simulink model "Advance_Battery_Cooling"  (R2021a)
settings: Solver=FixedStepAuto  StartTime=0.0  StopTime=1400  FixedStep=1  RelTol=1e-3
values from neighbouring files (symbols this model uses):
  Bc = 810.5328    [Battery_Cooling.m]
  c = 1350    [Battery_Cooling.m]
  Cell_length = 0.227    [Battery_Cooling.m]
  cell_volatge = Cell(:,2:3)    [Battery_Cooling.m]
  Cell_Width = 0.226    [Battery_Cooling.m]
  Cr = [0.0117,0.0085,0.0090 ... (first row only)    [Battery_Cooling.m]
  h_conv = 5    [Battery_Cooling.m]
  m_flow_air = BCP/(1350*(20.15-BPT_max))    [Battery_Cooling.m]
  Mb = 150.2    [Battery_Cooling.m]
  Np = 2    [Battery_Cooling.m]
  Ns = 96    [Battery_Cooling.m]
  Ri = 0.0023    [Battery_Cooling.m]
  SOC = [0;0.1;0.25;0.5;0.75;0.9;1]    [Battery_Cooling.m]
  T = [278.15;293.15;313.15]    [Battery_Cooling.m]
  Tamb = 293.15    [Battery_Cooling.m]
settings Model: Creator=LENOVO  LastModifiedBy=LENOVO

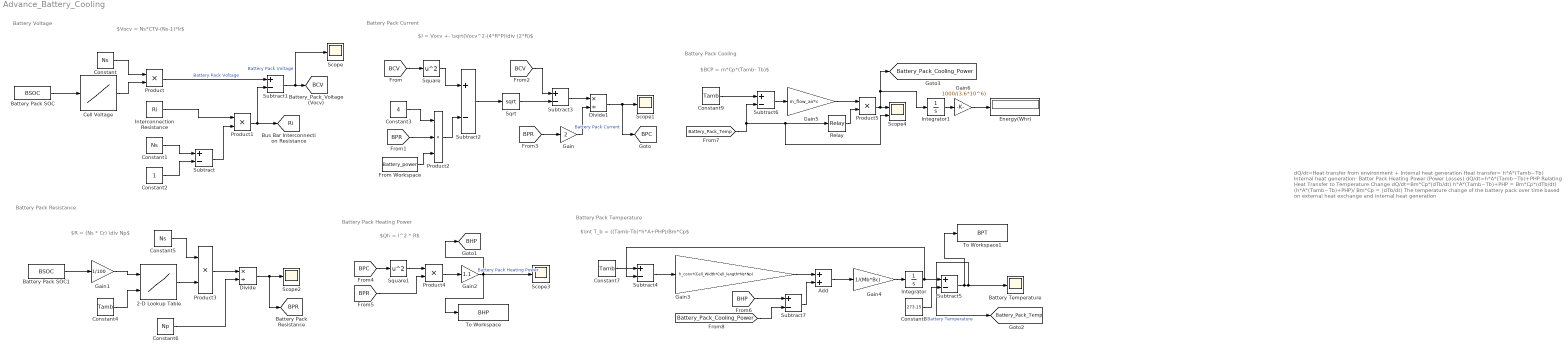
== system Advance_Battery_Cooling ==
  note: $BCP = m*Cp*(Tamb- Tb)$
  note: Battery Pack Cooling
  note: dQ/dt=Heat transfer from environment + Internal heat generation
      | Heat transfer= h*A*(Tamb​−Tb​)
      | Internal heat generation- Batter Pack Heating Power (Power Losses)
      | dQ​/dt=h*A*(Tamb​−Tb​)+PHP
      | Relating Heat Transfer to Temperature Change
      | dQ/dt​=Bm*Cp*(dTb​​/dt)
      | h*A*(Tamb​−Tb​)+PHP = Bm*Cp*(dTb​​/dt)
      | (h*A*(Tamb​−Tb​)+PHP)/ Bm*Cp = (dTb​​/dt)
      | The temperature change of the battery pack over time based on external heat exchange and internal heat generation
  note: Battery Pack Temperature
  note: $\int T_b = ((Tamb-Tb)*h*A+PHP)/Bm*Cp$
  note: Battery Pack Heating Power
  note: Battery Pack Current
  note: Battery Pack Resistance
  note: Battery Voltage
  note: $Vocv = Ns*CTV-(Ns-1)*Ir$
  note: $R = (Ns * Cr) \div Np$
  note: $Qh = I^2 * R$
  note: $I = Vocv +- \sqrt(Vocv^2-(4*R*P)\div (2*R)$
  2-D Lookup Table : Lookup_n-D  BreakpointsForDimension1=SOC  BreakpointsForDimension2=T  Table=Cr  InternalRulePriority=Speed  RndMeth=Simplest  InputSameDT=on
      settings: InputPortMap=u0,u1
  Add : Sum
  Battery Pack SOC : FromWorkspace  VariableName=BSOC
  Battery Pack SOC1 : FromWorkspace  VariableName=BSOC
  Battery Temperature : Scope
  Cell Voltage : Lookup_n-D  NumberOfTableDimensions=1  BreakpointsForDimension1=cell_volatge(:,2)  Table=cell_volatge(:,1)  InternalRulePriority=Speed  RndMeth=Simplest  InputSameDT=on
  Constant : Constant  Value=Ns
  Constant1 : Constant  Value=Ns
  Constant2 : Constant
  Constant3 : Constant  Value=4
  Constant4 : Constant  Value=Tamb
  Constant5 : Constant  Value=Ns
  Constant6 : Constant  Value=Np
  Constant7 : Constant  Value=Tamb
  Constant8 : Constant  Value=273.15
  Constant9 : Constant  Value=Tamb
  Divide : Product  Inputs=*/
  Divide1 : Product  Inputs=*/
  Energy(Whr) : Display
  From Workspace : FromWorkspace  VariableName=Battery_power
  Gain : Gain  Gain=2
  Gain1 : Gain  Gain=1/100
  Gain2 : Gain  Gain=1.1
  Gain3 : Gain  Gain=h_conv*(Cell_Width*Cell_length*Ns*Np)
  Gain4 : Gain  Gain=1/(Mb*Bc)
  Gain5 : Gain  Gain=m_flow_air*c
  Gain6 : Gain  Gain=1000/(3.6*10^6)
  Integrator : Integrator  InitialCondition=293
  Integrator1 : Integrator
  Interconnection Resistance : Constant  Value=Ri
  Product{,1,3..5} (5 alike) : Product
  Product2 : Product  Inputs=3
  Relay : Relay  OnSwitchValue=30  OffSwitchValue=20
  Scope{,1..3} (4 alike) : Scope
  Scope4 : Scope  NumInputPorts=2
  Sqrt : Sqrt  SaturateOnIntegerOverflow=on
  Square : Math  Operator=square  SaturateOnIntegerOverflow=on
  Square1 : Math  Operator=square  SaturateOnIntegerOverflow=on
  Subtract{,1..7} (8 alike) : Sum  Inputs=+-
  To Workspace : ToWorkspace  VariableName=BHP  SaveFormat=Timeseries  SampleTime=-1
  To Workspace1 : ToWorkspace  VariableName=BPT  SaveFormat=Timeseries  SampleTime=-1
  tag scope: BCV=global, BHP=global, BPC=global, BPR=global, Battery_Pack_Cooling_Power=global, Battery_Pack_Temp=global, Ri=global
  wires:
  Battery Pack SOC/1 -> Cell Voltage/1
  Constant/1 -> Product/1
  Cell Voltage/1 -> Product/2
  Constant1/1 -> Subtract/1
  Constant2/1 -> Subtract/2
  Interconnection Resistance/1 -> Product1/1
  Subtract/1 -> Product1/2
  Product/1 -> Subtract1/1  "Battery Pack Voltage"
  Product1/1 -> [Ri], Subtract1/2
  Subtract1/1 -> Scope/1, [BCV]  "Battery Pack Voltage"
  From Workspace/1 -> Product2/3
  [BPR] -> Product2/2
  Constant3/1 -> Product2/1
  [BCV] -> Square/1
  Product2/1 -> Subtract2/2
  Square/1 -> Subtract2/1
  Subtract2/1 -> Sqrt/1
  [BCV] -> Subtract3/1
  Constant4/1 -> 2-D Lookup Table/2
  Battery Pack SOC1/1 -> Gain1/1
  Gain1/1 -> 2-D Lookup Table/1
  Constant5/1 -> Product3/1
  2-D Lookup Table/1 -> Product3/2
  Product3/1 -> Divide/1
  Constant6/1 -> Divide/2
  Divide/1 -> [BPR], Scope2/1
  Sqrt/1 -> Subtract3/2
  Subtract3/1 -> Divide1/1
  Divide1/1 -> [BPC], Scope1/1  "Battery Pack Current"
  [BPR] -> Gain/1
  Gain/1 -> Divide1/2
  [BPC] -> Square1/1
  Square1/1 -> Product4/1
  [BPR] -> Product4/2
  Product4/1 -> Gain2/1
  Gain2/1 -> To Workspace/1, [BHP], Scope3/1  "Battery Pack Heating Power"
  Constant7/1 -> Subtract4/1
  Subtract4/1 -> Gain3/1
  Gain3/1 -> Add/1
  Add/1 -> Gain4/1
  Gain4/1 -> Integrator/1
  Integrator/1 -> Subtract4/2, Subtract5/1
  Constant8/1 -> Subtract5/2
  Subtract5/1 -> To Workspace1/1, [Battery_Pack_Temp], Battery Temperature/1  "Battery Temperature"
  Constant9/1 -> Subtract6/1
  [Battery_Pack_Temp] -> Scope4/2, Relay/1, Subtract6/2
  Subtract6/1 -> Gain5/1
  Gain5/1 -> Product5/1
  Relay/1 -> Product5/2
  Product5/1 -> [Battery_Pack_Cooling_Power], Integrator1/1, Scope4/1
  [BHP] -> Subtract7/1
  Subtract7/1 -> Add/2
  [Battery_Pack_Cooling_Power] -> Subtract7/2
  Integrator1/1 -> Gain6/1
  Gain6/1 -> Energy(Whr)/1
